simulink model "MotorSlider_RS_controlled"  (R2026a)
settings: Solver=FixedStepAuto  StopTime=1  FixedStep=0.0001
values from neighbouring files (symbols this model uses):
  den_C = [1, -1]    [Task2_run.m]
  num_C = [q0, q1]    [Task2_run.m]
libraries: fl_lib x27, nesl_utility x11, simulink x5, ee_lib x2
settings Model: Creator=lin-t  LastModifiedBy=strop
settings SimscapeCC: SimscapeNominalValues="[{\"value\":\"1\",\"unit\":\"A\"},{\"value\":\"1\",\"unit\":\"bar\"},{\"value\":\"1\",\"unit\":\"cm^2\"},{\"value\":\"1\",\"unit\":\"cm^3/s\"},{\"value\":\"1\",\"unit\":\"kJ/kg\"},{\"value\":\"1\",\"unit\":\"kW\"},{\"value\":\"1\",\"unit\":\"l\"},{\"value\":\"1\",\"unit\":\"N\"},{\"value\":\"1\",\"unit\":\"N*m\"},{\"value\":\"1\",\"unit\":\"V\"}]"  SimscapeLogType=none  SimscapeLogDataHistory=5000.0

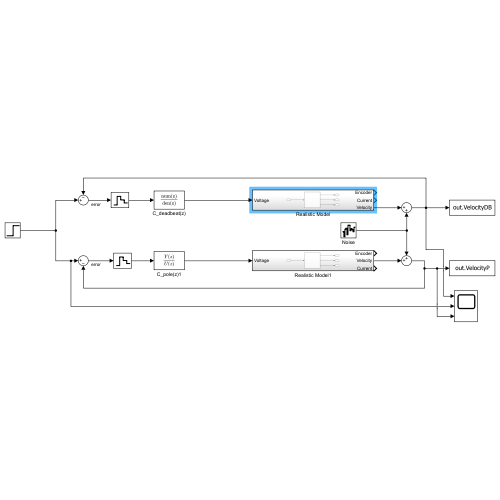
[thumbnail: Simulink's stored preview of the top-level diagram]
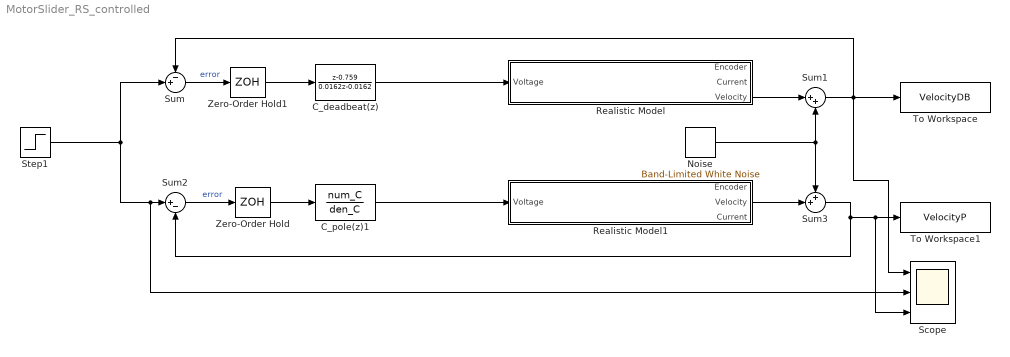
== system MotorSlider_RS_controlled ==
  C_deadbeat(z) : DiscreteTransferFcn  Numerator=[1 -0.759]  Denominator=[0.0162 -0.0162]
  C_pole(z)1 : DiscreteTransferFcn  Numerator=num_C  Denominator=den_C
  Noise : simulink/Sources/Band-Limited White Noise  Cov=noise_power  Ts=0.01  seed=[23341]
  Realistic Model : Subsystem
  Realistic Model1 : Subsystem
  Scope : Scope  NumInputPorts=3
      settings: ActiveDisplayYMinimum=-2836.3880775296698  ActiveDisplayYMaximum=4744.6648789244227
  Step1 : Step  Time=.3  FinalValue=velocityStep  SampleTime=0
  Sum : Sum  Inputs=-+|
  Sum1 : Sum  Inputs=|++
  Sum2 : Sum  Inputs=|+-
  Sum3 : Sum  Inputs=++|
  To Workspace : ToWorkspace  VariableName=VelocityDB  SaveFormat=Timeseries  SampleTime=-1
  To Workspace1 : ToWorkspace  VariableName=VelocityP  SaveFormat=Timeseries  SampleTime=-1
  Zero-Order Hold : ZeroOrderHold  SampleTime=0.02
  Zero-Order Hold1 : ZeroOrderHold  SampleTime=0.02
  wires:
  Sum1/1 -> Scope/1, Sum/1, To Workspace/1
  Realistic Model/3(Velocity) -> Sum1/1
  Noise/1 -> Sum1/2, Sum3/1
  Step1/1 -> Scope/2, Sum2/1, Sum/2
  Sum3/1 -> Scope/3, To Workspace1/1, Sum2/2
  C_pole(z)1/1 -> Realistic Model1/1(Voltage)
  Zero-Order Hold/1 -> C_pole(z)1/1
  Sum2/1 -> Zero-Order Hold/1  "error"
  Sum/1 -> Zero-Order Hold1/1  "error"
  Zero-Order Hold1/1 -> C_deadbeat(z)/1
  C_deadbeat(z)/1 -> Realistic Model/1(Voltage)
  Realistic Model1/2(Velocity) -> Sum3/2

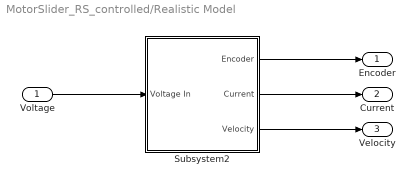
== system MotorSlider_RS_controlled/Realistic Model ==
  Voltage : Inport
  Subsystem2 : Subsystem
  Encoder : Outport
  Current : Outport  Port=2
  Velocity : Outport  Port=3
  wires:
  Subsystem2/2(Current) -> Current/1
  Subsystem2/3(Velocity) -> Velocity/1
  Subsystem2/1(Encoder) -> Encoder/1
  Voltage/1 -> Subsystem2/1(Voltage In)

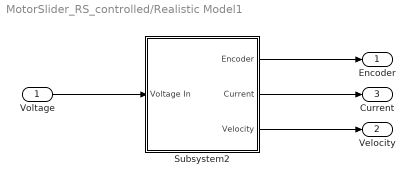
== system MotorSlider_RS_controlled/Realistic Model1 ==
  Voltage : Inport
  Subsystem2 : Subsystem
  Encoder : Outport
  Velocity : Outport  Port=2
  Current : Outport  Port=3
  wires:
  Subsystem2/2(Current) -> Current/1
  Subsystem2/3(Velocity) -> Velocity/1
  Subsystem2/1(Encoder) -> Encoder/1
  Voltage/1 -> Subsystem2/1(Voltage In)

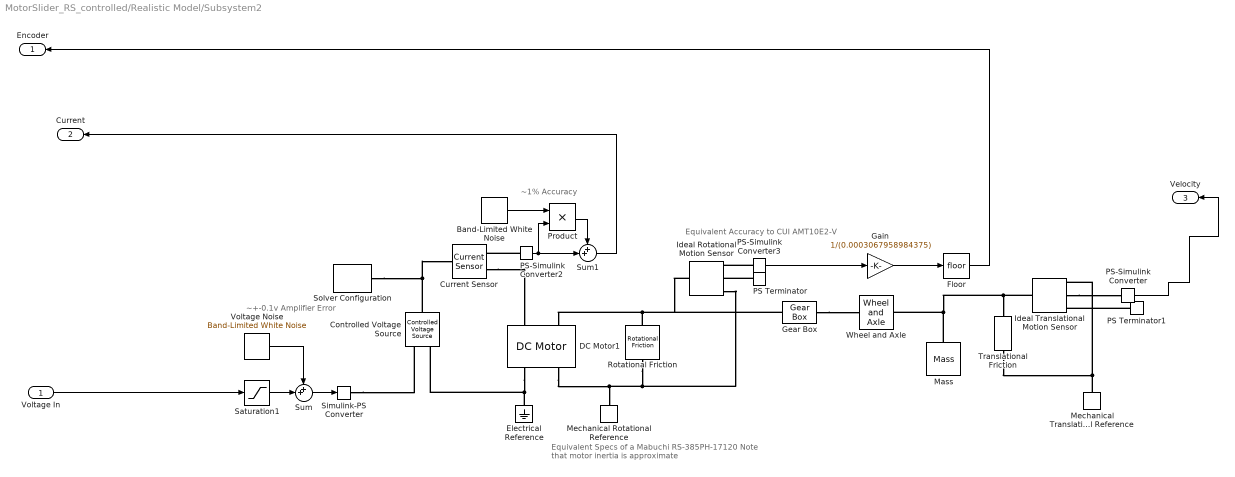
== system MotorSlider_RS_controlled/Realistic Model/Subsystem2 ==
  note: Equivalent Specs of a Mabuchi RS-385PH-17120
      | Note that motor inertia is approximate
  note: ~1% Accuracy
  note: Equivalent Accuracy to CUI AMT10E2-V
  note: ~+-0.1v Amplifier Error
  Voltage In : Inport
  Band-Limited White Noise : simulink/Sources/Band-Limited White Noise  Cov=[0.0000002]  Ts=0.01  seed=floor([rand() * 65535])
  Controlled Voltage Source : fl_lib/Electrical/Electrical Sources/Controlled Voltage Source
  Current Sensor : fl_lib/Electrical/Electrical Sensors/Current Sensor
  DC Motor1 : ee_lib/Electromechanical/Brushed Motors/DC Motor  field_option=ee.enum.field_option.pm  Rf=100 Ohm  Lf=1 H  Laf=0.15 H  If0=0 A  parameterization=ee.enum.dcparam_option.circuit_param  Ra=7.71 Ohm  La=12e-6 H  emf_or_torque=ee.enum.emf_or_torque.kv  Kv=0.0251 V/(rad/s)  Ki=6.876e-4 N*m/A  T_stall=0.24e-3 N*m  w_max=19100 rpm  w_rated=15000 rpm  P_rated=0.08 W  V_rated=1.5 V  lam_param=ee.enum.lam_param.damping  i_noload=0 A  V_i_noload=1.5 V  J=1.5e-6 kg*m^2  lam=0 N*m/(rad/s)  speed0=0 rpm  alpha=3.93e-3 1/K  Tmeas=25 degC  thermal_mass=100 J/K  initial_temperature=25 degC
  Electrical Reference : fl_lib/Electrical/Electrical Elements/Electrical Reference
  Floor : Rounding
  Gain : Gain  Gain=1/(0.0003067958984375)
  Gear Box : fl_lib/Mechanical/Mechanisms/Gear Box  ratio=3  t_in_specify=off  t_in_priority=None  t_in=0 N*m  t_in_nominal_specify=off  t_in_nominal_value=1  t_in_nominal_unit=N*m  t_out_specify=off  t_out_priority=None  t_out=0 N*m  t_out_nominal_specify=off  t_out_nominal_value=1  t_out_nominal_unit=N*m
  Ideal Rotational Motion Sensor : fl_lib/Mechanical/Mechanical Sensors/Ideal Rotational Motion Sensor  reference=foundation.enum.MeasurementReference.difference  acceleration_port=false  velocity_port=true  position_port=true  wrap_angle=simscape.enum.onoff.off  offset=0 rad
  Ideal Translational Motion Sensor : fl_lib/Mechanical/Mechanical Sensors/Ideal Translational Motion Sensor  reference=foundation.enum.MeasurementReference.difference  acceleration_port=false  velocity_port=true  position_port=true  offset=0 m
  Mass : fl_lib/Mechanical/Translational Elements/Mass  mass=1.5 kg  num_ports=foundation.enum.numPorts2.one  v_specify=off  v_priority=High  v=0 m/s  v_nominal_specify=off  v_nominal_value=1  v_nominal_unit=m/s  f_specify=off  f_priority=None  f=0 N  f_nominal_specify=off  f_nominal_value=1  f_nominal_unit=N
  Mechanical Rotational Reference : fl_lib/Mechanical/Rotational Elements/Mechanical Rotational Reference
  Mechanical Translational Reference : fl_lib/Mechanical/Translational Elements/Mechanical Translational Reference
  PS Terminator : fl_lib/Physical Signals/Sinks/PS Terminator
  PS Terminator1 : fl_lib/Physical Signals/Sinks/PS Terminator
  PS-Simulink Converter : nesl_utility/PS-Simulink Converter  PhysicalDomain=network_engine_domain  SubClassName=ps_output  LeftPortType=input  RightPortType=output  PseudoPeriodic=off  Frequencies=[]  VectorFormat=1-D array  Unit=inherit  AffineConversion=off
  PS-Simulink Converter2 : nesl_utility/PS-Simulink Converter  PhysicalDomain=network_engine_domain  SubClassName=ps_output  LeftPortType=input  RightPortType=output  PseudoPeriodic=off  Frequencies=[]  VectorFormat=1-D array  Unit=inherit  AffineConversion=off
  PS-Simulink Converter3 : nesl_utility/PS-Simulink Converter  PhysicalDomain=network_engine_domain  SubClassName=ps_output  LeftPortType=input  RightPortType=output  PseudoPeriodic=off  Frequencies=[]  VectorFormat=1-D array  Unit=inherit  AffineConversion=off
  Product : Product
  Rotational Friction : fl_lib/Mechanical/Rotational Elements/Rotational Friction  brkwy_trq=0.005 N*m  brkwy_vel=1e-9 rad/s  Col_trq=1e-9 N*m  visc_coef=2.148e-6 N*m/(rad/s)  w_specify=off  w_priority=None  w=0 rad/s  w_nominal_specify=off  w_nominal_value=1  w_nominal_unit=rad/s  t_specify=off  t_priority=None  t=0 N*m  t_nominal_specify=off  t_nominal_value=1  t_nominal_unit=N*m
  Saturation1 : Saturate  UpperLimit=15  LowerLimit=-15
  Simulink-PS Converter : nesl_utility/Simulink-PS Converter  PhysicalDomain=network_engine_domain  SubClassName=ps_input  LeftPortType=input  RightPortType=output  PseudoPeriodic=off  Frequencies=[]  NoiseDistribution=none  NoiseParameters=[]  Unit=1  AffineConversion=off  FilteringAndDerivatives=provide  SimscapeFilterOrder=1  InputFilterTimeConstant=0.001  UdotUserProvided=0
  Solver Configuration : nesl_utility/Solver Configuration  PhysicalDomain=network_engine_domain  SubClassName=solver  LeftPortType=input  RightPortType=generic  Tones=[]  Harmonics=[]  SimulateNoise=off  Profile=off  UseLocalSampling=off  EnableSwitchedLinearOptims=on  FrequencyDomain=off  UseCCode=off  RelTol=0.001  AbsTol=1e-06  MinStep=1e-09  ToWorkspace=off  RevertToSquareIcSolve=off  NumHomotopyIterations=100  PhasorMode=off  PhasorModeNumHarmonics=1  ConsistencySolver=NEWTON_FTOL  CanonicalOrdering=UNORDERED  OptimizeIntermediates=UNOPTIMIZED  IndexReductionMethod=DerivativeReplacement  DoDC=off  ResidualTolerance=1e-09  ConsistencyTolSource=GLOBAL  ConsistencyAbsTol=0.001  ConsistencyRelTol=0.001  ConsistencyTolFactor=0.001  UseLocalSolver=off  LocalSolverChoice=NE_BACKWARD_EULER_ADVANCER  ResolveIndetEquations=on  FunctionEvalNumThread=1  LocalSolverSampleTime=0.001  DoFixedCost=off  MaxNonlinIter=3  MaxModeIter=2  ComputeImpulses=off  ImpulseIterations=2  LinearAlgebra=auto  LinearAlgebraNumThread=0  EquationFormulation=NE_TIME_EF  DelaysMemoryBudget=1024  AutomaticFiltering=on  FilteringTimeConstant=0.001  PartitionStorageMethod=AS_NEEDED  PartitionMemoryBudget=1024  PartitionMethod=ROBUST  MultibodyUseLocalSolver=off  MultibodyLocalSolverChoice=ODE1  MultibodyLocalSolverSampleTime=0.001
  Sum : Sum  Inputs=++|
  Sum1 : Sum  Inputs=++|
  Translational Friction : fl_lib/Mechanical/Translational Elements/Translational Friction  brkwy_frc=0.2 N  brkwy_vel=0.01 m/s  Col_frc=0.05 N  visc_coef=0.05 N/(m/s)  v_specify=off  v_priority=None  v=0 m/s  v_nominal_specify=off  v_nominal_value=1  v_nominal_unit=m/s  f_specify=off  f_priority=None  f=0 N  f_nominal_specify=off  f_nominal_value=1  f_nominal_unit=N
  Voltage Noise : simulink/Sources/Band-Limited White Noise  Cov=[0.00001]  Ts=0.01  seed=floor([rand() * 65535])
  Wheel and Axle : fl_lib/Mechanical/Mechanisms/Wheel and Axle  R=0.5 cm  or=1  t_specify=off  t_priority=None  t=0 N*m  t_nominal_specify=off  t_nominal_value=1  t_nominal_unit=N*m  f_specify=off  f_priority=None  f=0 N  f_nominal_specify=off  f_nominal_value=1  f_nominal_unit=N
  Encoder : Outport
  Current : Outport  Port=2
  Velocity : Outport  Port=3
  wires:
  Sum1/1 -> Current/1
  PS-Simulink Converter2/1 -> Product/2, Sum1/2
  Saturation1/1 -> Sum/2
  Sum/1 -> Simulink-PS Converter/1
  Voltage In/1 -> Saturation1/1
  PS-Simulink Converter3/1 -> Gain/1
  Gain/1 -> Floor/1
  Band-Limited White Noise/1 -> Product/1
  Floor/1 -> Encoder/1
  Product/1 -> Sum1/1
  Voltage Noise/1 -> Sum/1
  PS-Simulink Converter/1 -> Velocity/1
  connections:
  Electrical Reference/LConn1 -- Controlled Voltage Source/RConn2 -- DC Motor1/RConn1
  Ideal Translational Motion Sensor/LConn1 -- Translational Friction/LConn1 -- Wheel and Axle/RConn1 -- Mass/LConn1
  PS Terminator1/LConn1 -- Ideal Translational Motion Sensor/RConn3
  Ideal Rotational Motion Sensor/RConn1 -- Rotational Friction/RConn1 -- DC Motor1/RConn2 -- Mechanical Rotational Reference/LConn1
  PS Terminator/LConn1 -- Ideal Rotational Motion Sensor/RConn2
  PS-Simulink Converter3/LConn1 -- Ideal Rotational Motion Sensor/RConn3
  Controlled Voltage Source/LConn1 -- Solver Configuration/RConn1 -- Current Sensor/LConn1
  Rotational Friction/LConn1 -- DC Motor1/LConn2 -- Ideal Rotational Motion Sensor/LConn1 -- Gear Box/LConn1
  Ideal Translational Motion Sensor/RConn2 -- PS-Simulink Converter/LConn1
  Mechanical Translational Reference/LConn1 -- Translational Friction/RConn1 -- Ideal Translational Motion Sensor/RConn1
  Simulink-PS Converter/RConn1 -- Controlled Voltage Source/RConn1
  Current Sensor/RConn2 -- DC Motor1/LConn1
  PS-Simulink Converter2/LConn1 -- Current Sensor/RConn1
  Gear Box/RConn1 -- Wheel and Axle/LConn1

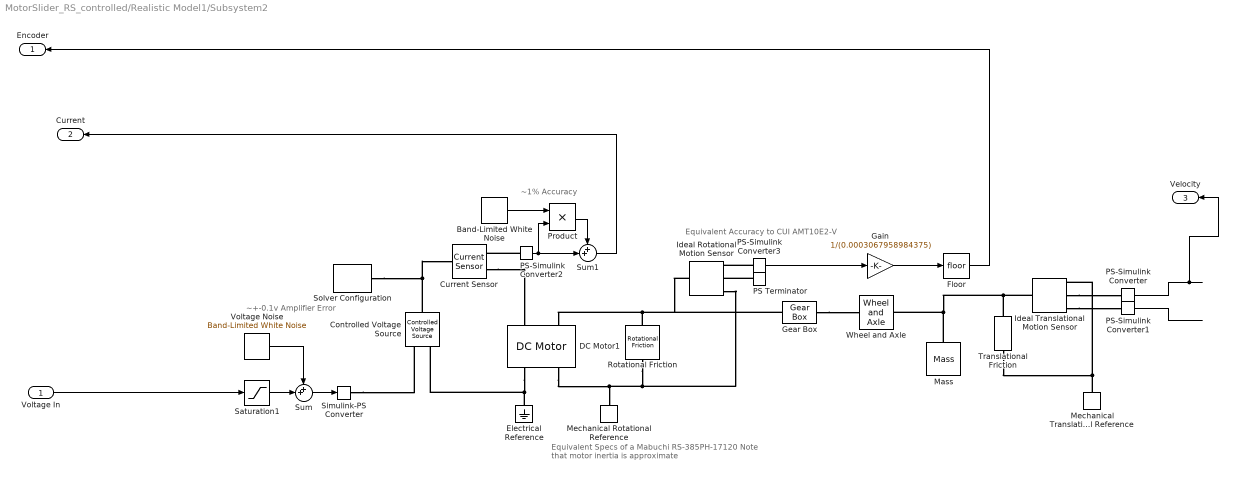
== system MotorSlider_RS_controlled/Realistic Model1/Subsystem2 ==
  note: Equivalent Specs of a Mabuchi RS-385PH-17120
      | Note that motor inertia is approximate
  note: ~1% Accuracy
  note: Equivalent Accuracy to CUI AMT10E2-V
  note: ~+-0.1v Amplifier Error
  Voltage In : Inport
  Band-Limited White Noise : simulink/Sources/Band-Limited White Noise  Cov=[0.0000002]  Ts=0.01  seed=floor([rand() * 65535])
  Controlled Voltage Source : fl_lib/Electrical/Electrical Sources/Controlled Voltage Source
  Current Sensor : fl_lib/Electrical/Electrical Sensors/Current Sensor
  DC Motor1 : ee_lib/Electromechanical/Brushed Motors/DC Motor  field_option=ee.enum.field_option.pm  Rf=100 Ohm  Lf=1 H  Laf=0.15 H  If0=0 A  parameterization=ee.enum.dcparam_option.circuit_param  Ra=7.71 Ohm  La=12e-6 H  emf_or_torque=ee.enum.emf_or_torque.kv  Kv=0.0251 V/(rad/s)  Ki=6.876e-4 N*m/A  T_stall=0.24e-3 N*m  w_max=19100 rpm  w_rated=15000 rpm  P_rated=0.08 W  V_rated=1.5 V  lam_param=ee.enum.lam_param.damping  i_noload=0 A  V_i_noload=1.5 V  J=1.5e-6 kg*m^2  lam=0 N*m/(rad/s)  speed0=0 rpm  alpha=3.93e-3 1/K  Tmeas=25 degC  thermal_mass=100 J/K  initial_temperature=25 degC
  Electrical Reference : fl_lib/Electrical/Electrical Elements/Electrical Reference
  Floor : Rounding
  Gain : Gain  Gain=1/(0.0003067958984375)
  Gear Box : fl_lib/Mechanical/Mechanisms/Gear Box  ratio=3  t_in_specify=off  t_in_priority=None  t_in=0 N*m  t_in_nominal_specify=off  t_in_nominal_value=1  t_in_nominal_unit=N*m  t_out_specify=off  t_out_priority=None  t_out=0 N*m  t_out_nominal_specify=off  t_out_nominal_value=1  t_out_nominal_unit=N*m
  Ideal Rotational Motion Sensor : fl_lib/Mechanical/Mechanical Sensors/Ideal Rotational Motion Sensor  reference=foundation.enum.MeasurementReference.difference  acceleration_port=false  velocity_port=true  position_port=true  wrap_angle=simscape.enum.onoff.off  offset=0 rad
  Ideal Translational Motion Sensor : fl_lib/Mechanical/Mechanical Sensors/Ideal Translational Motion Sensor  reference=foundation.enum.MeasurementReference.difference  acceleration_port=false  velocity_port=true  position_port=true  offset=0 m
  Mass : fl_lib/Mechanical/Translational Elements/Mass  mass=1.5 kg  num_ports=foundation.enum.numPorts2.one  v_specify=off  v_priority=High  v=0 m/s  v_nominal_specify=off  v_nominal_value=1  v_nominal_unit=m/s  f_specify=off  f_priority=None  f=0 N  f_nominal_specify=off  f_nominal_value=1  f_nominal_unit=N
  Mechanical Rotational Reference : fl_lib/Mechanical/Rotational Elements/Mechanical Rotational Reference
  Mechanical Translational Reference : fl_lib/Mechanical/Translational Elements/Mechanical Translational Reference
  PS Terminator : fl_lib/Physical Signals/Sinks/PS Terminator
  PS-Simulink Converter{,1..3} (4 alike) : nesl_utility/PS-Simulink Converter  PhysicalDomain=network_engine_domain  SubClassName=ps_output  LeftPortType=input  RightPortType=output  PseudoPeriodic=off  Frequencies=[]  VectorFormat=1-D array  Unit=inherit  AffineConversion=off
  Product : Product
  Rotational Friction : fl_lib/Mechanical/Rotational Elements/Rotational Friction  brkwy_trq=0.005 N*m  brkwy_vel=1e-9 rad/s  Col_trq=1e-9 N*m  visc_coef=2.148e-6 N*m/(rad/s)  w_specify=off  w_priority=None  w=0 rad/s  w_nominal_specify=off  w_nominal_value=1  w_nominal_unit=rad/s  t_specify=off  t_priority=None  t=0 N*m  t_nominal_specify=off  t_nominal_value=1  t_nominal_unit=N*m
  Saturation1 : Saturate  UpperLimit=15  LowerLimit=-15
  Simulink-PS Converter : nesl_utility/Simulink-PS Converter  PhysicalDomain=network_engine_domain  SubClassName=ps_input  LeftPortType=input  RightPortType=output  PseudoPeriodic=off  Frequencies=[]  NoiseDistribution=none  NoiseParameters=[]  Unit=1  AffineConversion=off  FilteringAndDerivatives=provide  SimscapeFilterOrder=1  InputFilterTimeConstant=0.001  UdotUserProvided=0
  Solver Configuration : nesl_utility/Solver Configuration  PhysicalDomain=network_engine_domain  SubClassName=solver  LeftPortType=input  RightPortType=generic  Tones=[]  Harmonics=[]  SimulateNoise=off  Profile=off  UseLocalSampling=off  EnableSwitchedLinearOptims=on  FrequencyDomain=off  UseCCode=off  RelTol=0.001  AbsTol=1e-06  MinStep=1e-09  ToWorkspace=off  RevertToSquareIcSolve=off  NumHomotopyIterations=100  PhasorMode=off  PhasorModeNumHarmonics=1  ConsistencySolver=NEWTON_FTOL  CanonicalOrdering=UNORDERED  OptimizeIntermediates=UNOPTIMIZED  IndexReductionMethod=DerivativeReplacement  DoDC=off  ResidualTolerance=1e-09  ConsistencyTolSource=GLOBAL  ConsistencyAbsTol=0.001  ConsistencyRelTol=0.001  ConsistencyTolFactor=0.001  UseLocalSolver=off  LocalSolverChoice=NE_BACKWARD_EULER_ADVANCER  ResolveIndetEquations=on  FunctionEvalNumThread=1  LocalSolverSampleTime=0.001  DoFixedCost=off  MaxNonlinIter=3  MaxModeIter=2  ComputeImpulses=off  ImpulseIterations=2  LinearAlgebra=auto  LinearAlgebraNumThread=0  EquationFormulation=NE_TIME_EF  DelaysMemoryBudget=1024  AutomaticFiltering=on  FilteringTimeConstant=0.001  PartitionStorageMethod=AS_NEEDED  PartitionMemoryBudget=1024  PartitionMethod=ROBUST  MultibodyUseLocalSolver=off  MultibodyLocalSolverChoice=ODE1  MultibodyLocalSolverSampleTime=0.001
  Sum : Sum  Inputs=++|
  Sum1 : Sum  Inputs=++|
  Translational Friction : fl_lib/Mechanical/Translational Elements/Translational Friction  brkwy_frc=0.2 N  brkwy_vel=0.01 m/s  Col_frc=0.05 N  visc_coef=0.05 N/(m/s)  v_specify=off  v_priority=None  v=0 m/s  v_nominal_specify=off  v_nominal_value=1  v_nominal_unit=m/s  f_specify=off  f_priority=None  f=0 N  f_nominal_specify=off  f_nominal_value=1  f_nominal_unit=N
  Voltage Noise : simulink/Sources/Band-Limited White Noise  Cov=[0.00001]  Ts=0.01  seed=floor([rand() * 65535])
  Wheel and Axle : fl_lib/Mechanical/Mechanisms/Wheel and Axle  R=0.5 cm  or=1  t_specify=off  t_priority=None  t=0 N*m  t_nominal_specify=off  t_nominal_value=1  t_nominal_unit=N*m  f_specify=off  f_priority=None  f=0 N  f_nominal_specify=off  f_nominal_value=1  f_nominal_unit=N
  Encoder : Outport
  Current : Outport  Port=2
  Velocity : Outport  Port=3
  wires:
  Sum1/1 -> Current/1
  PS-Simulink Converter2/1 -> Product/2, Sum1/2
  Saturation1/1 -> Sum/2
  Sum/1 -> Simulink-PS Converter/1
  Voltage In/1 -> Saturation1/1
  PS-Simulink Converter3/1 -> Gain/1
  Gain/1 -> Floor/1
  Band-Limited White Noise/1 -> Product/1
  Floor/1 -> Encoder/1
  Product/1 -> Sum1/1
  Voltage Noise/1 -> Sum/1
  PS-Simulink Converter1/1 -> ?
  PS-Simulink Converter/1 -> Velocity/1
  connections:
  Electrical Reference/LConn1 -- Controlled Voltage Source/RConn2 -- DC Motor1/RConn1
  Translational Friction/LConn1 -- Ideal Translational Motion Sensor/LConn1 -- Wheel and Axle/RConn1 -- Mass/LConn1
  Ideal Translational Motion Sensor/RConn3 -- PS-Simulink Converter1/LConn1
  Ideal Rotational Motion Sensor/RConn1 -- Rotational Friction/RConn1 -- DC Motor1/RConn2 -- Mechanical Rotational Reference/LConn1
  PS Terminator/LConn1 -- Ideal Rotational Motion Sensor/RConn2
  PS-Simulink Converter3/LConn1 -- Ideal Rotational Motion Sensor/RConn3
  Controlled Voltage Source/LConn1 -- Solver Configuration/RConn1 -- Current Sensor/LConn1
  Rotational Friction/LConn1 -- DC Motor1/LConn2 -- Ideal Rotational Motion Sensor/LConn1 -- Gear Box/LConn1
  Ideal Translational Motion Sensor/RConn2 -- PS-Simulink Converter/LConn1
  Mechanical Translational Reference/LConn1 -- Translational Friction/RConn1 -- Ideal Translational Motion Sensor/RConn1
  Simulink-PS Converter/RConn1 -- Controlled Voltage Source/RConn1
  Current Sensor/RConn2 -- DC Motor1/LConn1
  PS-Simulink Converter2/LConn1 -- Current Sensor/RConn1
  Gear Box/RConn1 -- Wheel and Axle/LConn1
